simulink subsystem "MPC9_nlpsol"  (R2022b)
settings: Solver=VariableStepAuto  StartTime=0.0  StopTime=10.0  RelTol=1e-3
undefined symbols (not defined in the file): param_MPC9, param_robot, param_traj_data, param_weight_init
settings Model: Creator=emu  LastModifiedBy=emu
settings OptimizationCC: ReuseModelBlockBuffer=on

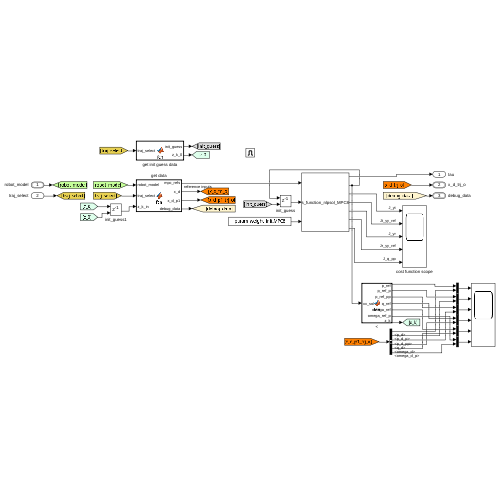
[thumbnail: Simulink's stored preview of the top-level diagram]
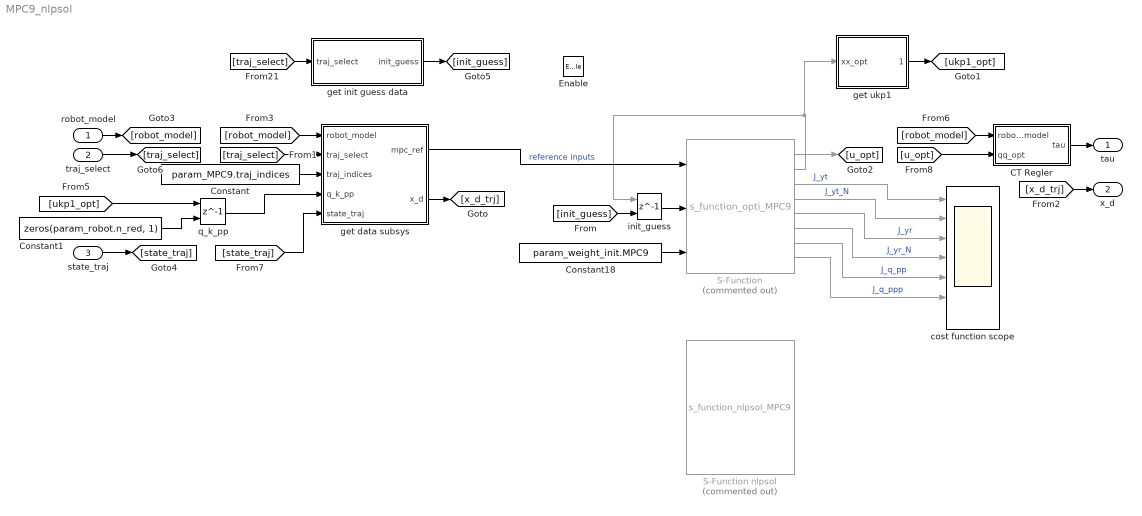
== system MPC9_nlpsol ==
  robot_model : Inport  OutDataTypeStr=Bus: robot_model
  traj_select : Inport  Port=2
  state_traj : Inport  Port=3  OutDataTypeStr=Bus: state_traj_bus
  Enable : EnablePort
  CT Regler : MATLAB Function  TreatAsAtomicUnit=on
  Constant : Constant  Value=param_MPC9.traj_indices
  Constant1 : Constant  Value=zeros(param_robot.n_red, 1)  VectorParams1D=off
  Constant18 : Constant  Value=param_weight_init.MPC9  VectorParams1D=off
  S-Function : S-Function  Commented=on  FunctionName=s_function_opti_MPC9  SFunctionModules='MPC9'  SFunctionDeploymentMode=off  EnableBusSupport=off
  S-Function nlpsol : S-Function  Commented=on  FunctionName=s_function_nlpsol_MPC9  Parameters='s_functions/fr3_no_hand_6dof/MPC9.casadi', 'MPC9'  SFunctionModules='MPC9'  SFunctionDeploymentMode=off  EnableBusSupport=off
  cost function scope : Scope  NumInputPorts=7
  get data subsys : Subsystem
  get init guess data : MATLAB Function  TreatAsAtomicUnit=on
  get ukp1 : MATLAB Function  TreatAsAtomicUnit=on
  init_guess : Delay  DelayLength=1  InitialConditionSource=Input port  InitialCondition=1
      settings: InputPortMap=u0,p4
  q_k_pp : Delay  DelayLength=1  InitialConditionSource=Input port  InitialCondition=1
      settings: InputPortMap=u0,p4
  tau : Outport
  x_d : Outport  Port=2  OutDataTypeStr=Bus: x_d
  wires:
  [state_traj] -> get data subsys/5(state_traj)
  state_traj/1 -> [state_traj]
  CT Regler/1(tau) -> tau/1
  [u_opt] -> CT Regler/2(qq_opt)
  S-Function/1 -> [u_opt]
  [robot_model] -> CT Regler/1(robot_model)
  S-Function/4 -> cost function scope/2  "J_yt_N"
  S-Function/2 -> init_guess/1, get ukp1/1(xx_opt)
  Constant18/1 -> S-Function/3
  [init_guess] -> init_guess/2
  S-Function/3 -> cost function scope/1  "J_yt"
  robot_model/1 -> [robot_model]
  [traj_select] -> get init guess data/1(traj_select)
  get init guess data/1(init_guess) -> [init_guess]
  init_guess/1 -> S-Function/2
  S-Function/5 -> cost function scope/3  "J_yr"
  traj_select/1 -> [traj_select]
  S-Function/6 -> cost function scope/4  "J_yr_N"
  S-Function/7 -> cost function scope/5  "J_q_pp"
  S-Function/8 -> cost function scope/6  "J_q_ppp"
  [traj_select] -> get data subsys/2(traj_select)
  [robot_model] -> get data subsys/1(robot_model)
  Constant/1 -> get data subsys/3(traj_indices)
  get data subsys/1(mpc_ref) -> S-Function/1  "reference inputs"
  [x_d_trj] -> x_d/1
  get data subsys/2(x_d) -> [x_d_trj]
  Constant1/1 -> q_k_pp/2
  [ukp1_opt] -> q_k_pp/1
  q_k_pp/1 -> get data subsys/4(q_k_pp)
  get ukp1/1(ukp1_opt) -> [ukp1_opt]

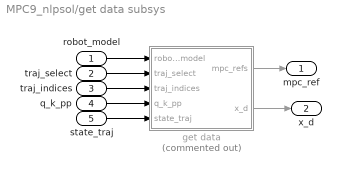
== system MPC9_nlpsol/get data subsys ==
  robot_model : Inport  OutDataTypeStr=Bus: robot_model
  traj_select : Inport  Port=2
  traj_indices : Inport  Port=3
  q_k_pp : Inport  Port=4
  state_traj : Inport  Port=5  OutDataTypeStr=Bus: state_traj_bus
  get data : MATLAB Function  Commented=on  TreatAsAtomicUnit=on
  mpc_ref : Outport
  x_d : Outport  Port=2  OutDataTypeStr=Bus: x_d
  wires:
  q_k_pp/1 -> get data/4(q_k_pp)
  robot_model/1 -> get data/1(robot_model)
  get data/2(x_d) -> x_d/1
  traj_select/1 -> get data/2(traj_select)
  traj_indices/1 -> get data/3(traj_indices)
  get data/1(mpc_refs) -> mpc_ref/1
  state_traj/1 -> get data/5(state_traj)

== matlab function MPC9_nlpsol/get ukp1 ==
  data: xx_opt input; ukp1_opt output; param_robot parameter; param_MPC9 parameter
function ukp1_opt = fcn(xx_opt, param_robot, param_MPC9)

N_MPC = param_MPC9.N;
n_red = param_robot.n_red;
ukp1_opt = xx_opt(1+N_MPC*n_red : (N_MPC+1)*n_red)';

== matlab function MPC9_nlpsol/get init guess data ==
  data: traj_select input; param_MPC9_init_guess parameter; init_guess output
function init_guess   = fcn(traj_select, param_MPC9_init_guess)

init_guess = param_MPC9_init_guess.init_guess(traj_select,:);

== matlab function MPC9_nlpsol/CT Regler ==
  data: robot_model input Bus: robot_model; tau output; qq_opt input; param_robot parameter
function tau = fcn(robot_model, qq_opt, param_robot)

n = param_robot.n_DOF;

if size(qq_opt, 2) ~= 0 && size(qq_opt, 1) ~= 1
    n_indices = param_robot.n_indices;
    q_d_pp = qq_opt;
    M = robot_model.M;      % inertia matrix
    g = robot_model.g;
    C_rnea = robot_model.C_rnea; % C_rnea(q, q_p) = C(q, q_p)q_p + g(q) = n(q, q_p)
    
    q_pp = zeros(n,1);
    q_pp(n_indices) = q_d_pp;
    
    tau = M*q_pp + C_rnea - g;
else
    tau = zeros(n,1);
end

== matlab function MPC9_nlpsol/get data subsys/get data ==
  settings: updateMethod=DISCRETE  sampleTime=param_global.Ta
  data: mpc_refs output; robot_model input Bus: robot_model; traj_select input; traj_indices input; param_traj_data parameter; x_d output Bus: x_d; param_robot parameter; q_k_pp input; state_traj input Bus: state_traj_bus
function [mpc_refs, x_d]  = fcn(robot_model, traj_select, traj_indices, param_traj_data, param_robot, q_k_pp, state_traj)
persistent cnt;
persistent run_flag;

if(isempty(cnt))
    cnt = 1;
    run_flag = 0;
end

n_indices = param_robot.n_indices;
traj_indices = traj_indices + (cnt-1);

% Parameters
q    = robot_model.q;      % generalized coordinates
q_p  = robot_model.q_p;  % time derivative of generalized coordinates

x_k = [q(n_indices);q_p(n_indices);q_k_pp];

% Assemble vector of recieved output measurements
p_d     = param_traj_data.p_d(   1:3, traj_indices, traj_select);
q_d     = param_traj_data.q_d(   1:4, traj_indices, traj_select);

y_d = [p_d; q_d];

%% Reference out
mpc_refs = [x_k(:); y_d(:)];

%% Offline Trajectory out
x_d.p_d            = param_traj_data.p_d(           :,    cnt, traj_select);
x_d.p_d_p          = param_traj_data.p_d_p(         :,    cnt, traj_select);
x_d.p_d_pp         = param_traj_data.p_d_pp(        :,    cnt, traj_select);
x_d.Phi_d          = param_traj_data.Phi_d(         :,    cnt, traj_select);
x_d.Phi_d_p        = param_traj_data.Phi_d_p(       :,    cnt, traj_select);
x_d.Phi_d_pp       = param_traj_data.Phi_d_pp(      :,    cnt, traj_select);
x_d.R_d            = param_traj_data.R_d(           :, :, cnt, traj_select);
x_d.q_d            = param_traj_data.q_d(           :,    cnt, traj_select);
x_d.q_d_p          = param_traj_data.q_d_p(         :,    cnt, traj_select);
x_d.q_d_pp         = param_traj_data.q_d_pp(        :,    cnt, traj_select);
x_d.omega_d        = param_traj_data.omega_d(       :,    cnt, traj_select);
x_d.omega_d_p      = param_traj_data.omega_d_p(     :,    cnt, traj_select);
x_d.alpha_d        = param_traj_data.alpha_d(       :,    cnt, traj_select);
x_d.alpha_d_p      = param_traj_data.alpha_d_p(     :,    cnt, traj_select);
x_d.alpha_d_pp     = param_traj_data.alpha_d_pp(    :,    cnt, traj_select);
x_d.rot_ax_d       = param_traj_data.rot_ax_d(      :,    cnt, traj_select);
x_d.alpha_d_offset = param_traj_data.alpha_d_offset(:,    cnt, traj_select);
x_d.q_d_rel        = param_traj_data.q_d_rel(       :,    cnt, traj_select);

[run_flag, cnt] = update_traj_cnt(state_traj, run_flag, cnt, param_traj_data.N);
